simulink model "noisyAccSensor"  (R2018a)
settings: Solver=ode4  StartTime=0.0  StopTime=50  FixedStep=0.001  RelTol=1e-3
undefined symbols (not defined in the file): omega
libraries: simulink x1
settings Model: Creator=Amir  LastModifiedBy=Amir
settings DebuggingCC: LibraryContextMissingDiagnostic=warning
settings SFSimCC: SimUseLocalCustomCode=on
settings RTWCC: RTWUseLocalCustomCode=on

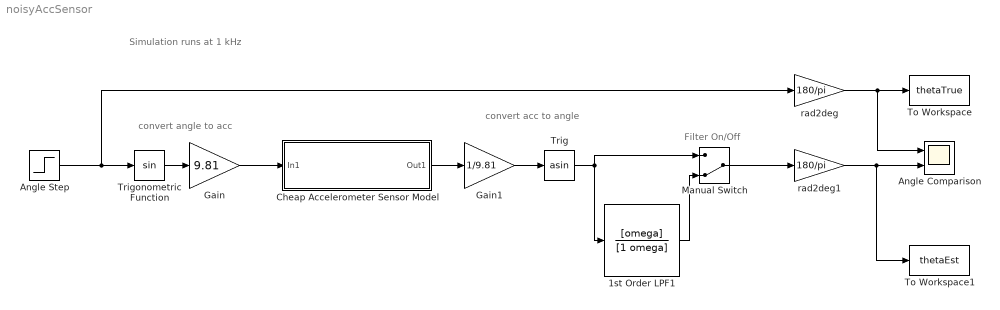
== system noisyAccSensor ==
  note: convert acc to angle
  note: convert angle to acc
  note: Simulation runs at 1 kHz
  note: Filter On/Off
  1st Order LPF1 : TransferFcn  Numerator=[omega]  Denominator=[1 omega]
  Angle Comparison : Scope  NumInputPorts=2
  Angle Step : Step  Time=25  After=pi/4  SampleTime=0
  Cheap Accelerometer Sensor Model : Subsystem
  Gain : Gain  Gain=9.81
  Gain1 : Gain  Gain=1/9.81
  Manual Switch : ManualSwitch  CurrentSetting=0
  To Workspace : ToWorkspace  VariableName=thetaTrue  SampleTime=-1
  To Workspace1 : ToWorkspace  VariableName=thetaEst  SampleTime=-1
  Trig : Trigonometry  Operator=asin
  Trigonometric Function : Trigonometry
  rad2deg : Gain  Gain=180/pi
  rad2deg1 : Gain  Gain=180/pi
  wires:
  Trigonometric Function/1 -> Gain/1
  Cheap Accelerometer Sensor Model/1(Out1) -> Gain1/1
  Gain/1 -> Cheap Accelerometer Sensor Model/1(In1)
  Angle Step/1 -> rad2deg/1, Trigonometric Function/1
  Gain1/1 -> Trig/1
  Trig/1 -> 1st Order LPF1/1, Manual Switch/1
  rad2deg/1 -> Angle Comparison/1, To Workspace/1
  rad2deg1/1 -> To Workspace1/1, Angle Comparison/2
  Manual Switch/1 -> rad2deg1/1
  1st Order LPF1/1 -> Manual Switch/2

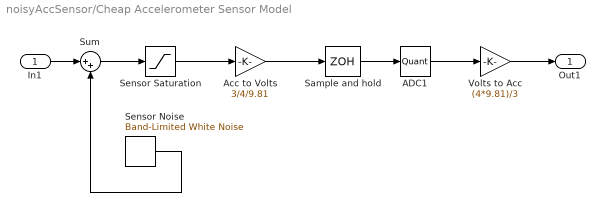
== system noisyAccSensor/Cheap Accelerometer Sensor Model ==
  In1 : Inport
  ADC1 : Quantizer  QuantizationInterval=3/(2^16-1)
  Acc to Volts : Gain  Gain=3/4/9.81
  Sample and hold : ZeroOrderHold  SampleTime=0.02
  Sensor Noise : simulink/Sources/Band-Limited White Noise  Cov=0.001  Ts=0.001  seed=[23341]
  Sensor Saturation : Saturate  UpperLimit=4*9.81  LowerLimit=-4*9.81
  Sum : Sum  Inputs=|++
  Volts to Acc : Gain  Gain=(4*9.81)/3
  Out1 : Outport
  wires:
  Sensor Noise/1 -> Sum/2
  ADC1/1 -> Volts to Acc/1
  In1/1 -> Sum/1
  Sensor Saturation/1 -> Acc to Volts/1
  Acc to Volts/1 -> Sample and hold/1
  Volts to Acc/1 -> Out1/1
  Sum/1 -> Sensor Saturation/1
  Sample and hold/1 -> ADC1/1
